simulink model "PID_Controller_sim"  (R2023a)
settings: Solver=VariableStepAuto  StartTime=0.0  StopTime=20  RelTol=1e-3
values from neighbouring files (symbols this model uses):
  c = 2050    [PID_Controller.m]    (also in set_Fun.m)
  ks = 60000    [PID_Controller.m]    (also in set_Fun.m)
  kt = 362000    [PID_Controller.m]    (also in set_Fun.m)
  ms = 1173    [PID_Controller.m]    (also in set_Fun.m)
  mu = 152.1    [PID_Controller.m]    (also in set_Fun.m)
  num_y1 = num(1,:)    [PID_Controller.m]
  num_y2 = num(2,:)    [PID_Controller.m]
  num_y3 = num(3,:)    [PID_Controller.m]
undefined symbols (not defined in the file or in its folder): den
libraries: slpidlib x5
settings Model: Creator=Administrator  LastModifiedBy=Administrator

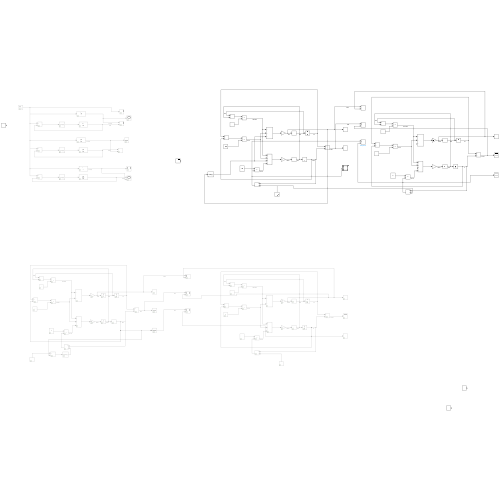
[thumbnail: Simulink's stored preview of the top-level diagram]
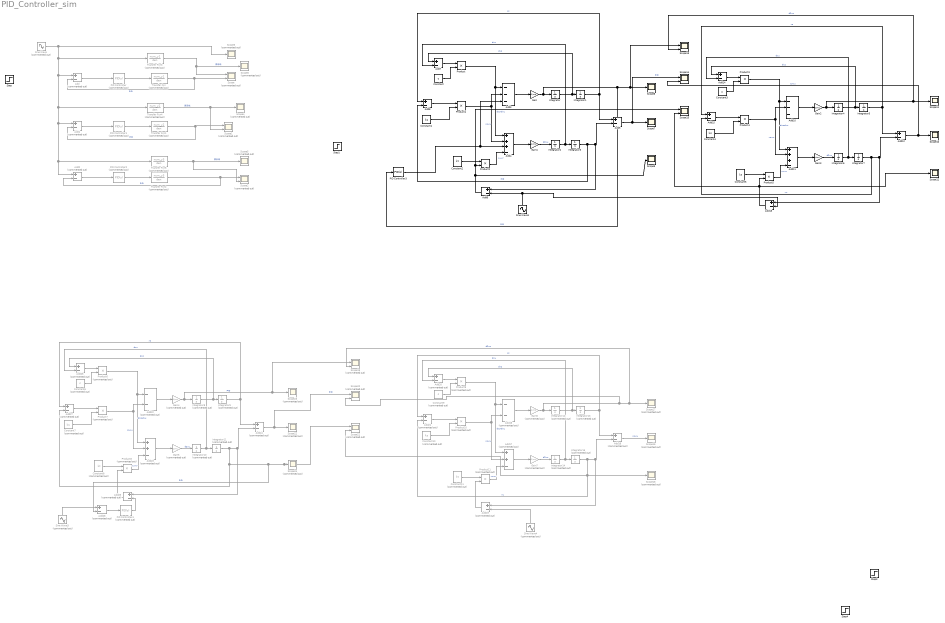
== system PID_Controller_sim ==
  Add{,1..2,18..21,24..28} (12 alike) : Sum  Commented=on  Inputs=+-
  Add10 : Sum  Inputs=---
  Add11 : Sum  Inputs=+++-
  Add{5..8,12..15} (8 alike) : Sum  Inputs=+-
  Add16 : Sum  Commented=on  Inputs=--
  Add17 : Sum  Commented=on  Inputs=++-
  Add22 : Sum  Commented=on  Inputs=--
  Add23 : Sum  Commented=on  Inputs=++-
  Add3 : Sum  Inputs=---
  Add4 : Sum  Inputs=+++-
  Constant : Constant  Value=c
  Constant1 : Constant  Value=ks
  Constant10 : Constant  Commented=on  Value=ks
  Constant11 : Constant  Commented=on  Value=kt
  Constant2 : Constant  Value=kt
  Constant3 : Constant  Value=c
  Constant4 : Constant  Value=ks
  Constant5 : Constant  Value=kt
  Constant6 : Constant  Commented=on  Value=c
  Constant7 : Constant  Commented=on  Value=ks
  Constant8 : Constant  Commented=on  Value=kt
  Constant9 : Constant  Commented=on  Value=c
  Gain : Gain  Gain=1/ms
  Gain1 : Gain  Gain=1/mu
  Gain2 : Gain  Gain=1/ms
  Gain3 : Gain  Gain=1/mu
  Gain4 : Gain  Commented=on  Gain=1/ms
  Gain5 : Gain  Commented=on  Gain=1/mu
  Gain6 : Gain  Commented=on  Gain=1/ms
  Gain7 : Gain  Commented=on  Gain=1/mu
  Integrator{,1..7} (8 alike) : Integrator
  Integrator{8..15} (8 alike) : Integrator  Commented=on
  PID Controller : slpidlib/PID Controller  Commented=on  Controller=PID  Form=Parallel  TimeDomain=Continuous-time  UseExternalTs=off  SampleTime=-1  IntegratorMethod=Forward Euler  FilterMethod=Forward Euler  ControllerParametersSource=internal  P=0.544393537633049  I=228.313262527094  UseKiTs=off  D=4.11995694275818e-05  N=8640.6528392362  UseFilter=on  TunerSelectOption=Transfer Function Based (PID Tuner App)  InitialConditionSource=internal  InitialConditionForIntegrator=0  InitialConditionForFilter=0  DifferentiatorICPrevScaledInput=0  ExternalReset=none  TrackingMode=off  Kt=1  LimitOutput=off  SatLimitsSource=internal  UpperSaturationLimit=inf  LowerSaturationLimit=-inf  LinearizeAsGain=on  AntiWindupMode=none  Kb=1  LimitIntegrator=off  UpperIntegratorSaturationLimit=inf  LowerIntegratorSaturationLimit=-inf  POutMin=[]  POutMax=[]  IOutMin=[]  IOutMax=[]  DOutMin=[]  DOutMax=[]  NOutMin=[]  NOutMax=[]  SumOutMin=[]  SumOutMax=[]  SaturationOutMin=[]  SaturationOutMax=[]  PParamMin=[]  PParamMax=[]  IParamMin=[]  IParamMax=[]  DParamMin=[]  DParamMax=[]  NParamMin=[]  NParamMax=[]  KbParamMin=[]  KbParamMax=[]  KtParamMin=[]  KtParamMax=[]  KbOutMin=[]  KbOutMax=[]  KtOutMin=[]  KtOutMax=[]  IntegratorOutMin=[]  IntegratorOutMax=[]  FilterOutMin=[]  FilterOutMax=[]  SumI1OutMin=[]  SumI1OutMax=[]  SumI2OutMin=[]  SumI2OutMax=[]  SumI3OutMin=[]  SumI3OutMax=[]  SumI4OutMin=[]  SumI4OutMax=[]  SumDOutMin=[]  SumDOutMax=[]  DifferentiatorOutMin=[]  DifferentiatorOutMax=[]  FilterDiffOutCoefMin=[]  FilterDiffOutCoefMax=[]  ReciprocalOutMin=[]  ReciprocalOutMax=[]  SumDenOutMin=[]  SumDenOutMax=[]  SumNumOutMin=[]  SumNumOutMax=[]  DivideOutMin=[]  DivideOutMax=[]  UdiffTsProdOutMin=[]  UdiffTsProdOutMax=[]  NTsProdOutMin=[]  NTsProdOutMax=[]  UintegralTsProdOutMin=[]  UintegralTsProdOutMax=[]  UngainTsProdOutMin=[]  UngainTsProdOutMax=[]  ClampingZeroOutDataTypeStr=Inherit: Inherit via back propagation  ClampingZeroOutMin=[]  ClampingZeroOutMax=[]  FilterDenConstantOutDataTypeStr=Inherit: Inherit via back propagation  FilterDenConstantOutMin=[]  FilterDenConstantOutMax=[]  PCopyOutDataTypeStr=Inherit: Inherit via back propagation  PCopyOutMin=[]  PCopyOutMax=[]  NCopyOutDataTypeStr=Inherit: Inherit via back propagation  NCopyOutMin=[]  NCopyOutMax=[]  IntegratorContinuousStateAttributes=''  IntegratorStateMustResolveToSignalObject=off  IntegratorRTWStateStorageClass=Auto  FilterContinuousStateAttributes=''  FilterStateMustResolveToSignalObject=off  FilterRTWStateStorageClass=Auto  ParallelPVariant=InternalParameters  IdealPVariant=Disabled  IVariant=InternalParameters  DVariant=InternalParameters  IntegratorVariant=Continuous  SatVariant=Disabled  AWVariant=Passthrough  PCopyVariant=Disabled  TRVariant=Disabled  FdbkBlocksVariant=Forward  IdealPFdbkVariant=Disabled  SatFdbkVariant=Disabled  DerivativeFilterVariant=ContFilter  NVariant=InternalParameters  NCopyVariant=Disabled  FilterICVariant=InternalICsFilter  IntegratorICVariant=InternalICs  ExternalResetVariant=Disabled  TRSumVariant=Passthrough  SumFdbkVariant=Disabled  SumVariant=Sum_PID  TsampFilterVariant=InternalTs  TsampNgainVariant=Passthrough  TsampIntegralVariant=Disabled_SignalSpec  ExternalSaturationOutDataTypeStr=Inherit: Same as second input
  PID Controller1 : slpidlib/PID Controller  Commented=on  Controller=PID  Form=Parallel  TimeDomain=Continuous-time  UseExternalTs=off  SampleTime=-1  IntegratorMethod=Forward Euler  FilterMethod=Forward Euler  ControllerParametersSource=internal  P=-344.974819520367  I=-34693.2038324327  UseKiTs=off  D=-0.842159264151759  N=11254.9743438156  UseFilter=on  TunerSelectOption=Transfer Function Based (PID Tuner App)  InitialConditionSource=internal  InitialConditionForIntegrator=0  InitialConditionForFilter=0  DifferentiatorICPrevScaledInput=0  ExternalReset=none  TrackingMode=off  Kt=1  LimitOutput=off  SatLimitsSource=internal  UpperSaturationLimit=inf  LowerSaturationLimit=-inf  LinearizeAsGain=on  AntiWindupMode=none  Kb=1  LimitIntegrator=off  UpperIntegratorSaturationLimit=inf  LowerIntegratorSaturationLimit=-inf  POutMin=[]  POutMax=[]  IOutMin=[]  IOutMax=[]  DOutMin=[]  DOutMax=[]  NOutMin=[]  NOutMax=[]  SumOutMin=[]  SumOutMax=[]  SaturationOutMin=[]  SaturationOutMax=[]  PParamMin=[]  PParamMax=[]  IParamMin=[]  IParamMax=[]  DParamMin=[]  DParamMax=[]  NParamMin=[]  NParamMax=[]  KbParamMin=[]  KbParamMax=[]  KtParamMin=[]  KtParamMax=[]  KbOutMin=[]  KbOutMax=[]  KtOutMin=[]  KtOutMax=[]  IntegratorOutMin=[]  IntegratorOutMax=[]  FilterOutMin=[]  FilterOutMax=[]  SumI1OutMin=[]  SumI1OutMax=[]  SumI2OutMin=[]  SumI2OutMax=[]  SumI3OutMin=[]  SumI3OutMax=[]  SumI4OutMin=[]  SumI4OutMax=[]  SumDOutMin=[]  SumDOutMax=[]  DifferentiatorOutMin=[]  DifferentiatorOutMax=[]  FilterDiffOutCoefMin=[]  FilterDiffOutCoefMax=[]  ReciprocalOutMin=[]  ReciprocalOutMax=[]  SumDenOutMin=[]  SumDenOutMax=[]  SumNumOutMin=[]  SumNumOutMax=[]  DivideOutMin=[]  DivideOutMax=[]  UdiffTsProdOutMin=[]  UdiffTsProdOutMax=[]  NTsProdOutMin=[]  NTsProdOutMax=[]  UintegralTsProdOutMin=[]  UintegralTsProdOutMax=[]  UngainTsProdOutMin=[]  UngainTsProdOutMax=[]  ClampingZeroOutDataTypeStr=Inherit: Inherit via back propagation  ClampingZeroOutMin=[]  ClampingZeroOutMax=[]  FilterDenConstantOutDataTypeStr=Inherit: Inherit via back propagation  FilterDenConstantOutMin=[]  FilterDenConstantOutMax=[]  PCopyOutDataTypeStr=Inherit: Inherit via back propagation  PCopyOutMin=[]  PCopyOutMax=[]  NCopyOutDataTypeStr=Inherit: Inherit via back propagation  NCopyOutMin=[]  NCopyOutMax=[]  IntegratorContinuousStateAttributes=''  IntegratorStateMustResolveToSignalObject=off  IntegratorRTWStateStorageClass=Auto  FilterContinuousStateAttributes=''  FilterStateMustResolveToSignalObject=off  FilterRTWStateStorageClass=Auto  ParallelPVariant=InternalParameters  IdealPVariant=Disabled  IVariant=InternalParameters  DVariant=InternalParameters  IntegratorVariant=Continuous  SatVariant=Disabled  AWVariant=Passthrough  PCopyVariant=Disabled  TRVariant=Disabled  FdbkBlocksVariant=Forward  IdealPFdbkVariant=Disabled  SatFdbkVariant=Disabled  DerivativeFilterVariant=ContFilter  NVariant=InternalParameters  NCopyVariant=Disabled  FilterICVariant=InternalICsFilter  IntegratorICVariant=InternalICs  ExternalResetVariant=Disabled  TRSumVariant=Passthrough  SumFdbkVariant=Disabled  SumVariant=Sum_PID  TsampFilterVariant=InternalTs  TsampNgainVariant=Passthrough  TsampIntegralVariant=Disabled_SignalSpec  ExternalSaturationOutDataTypeStr=Inherit: Same as second input
  PID Controller2 : slpidlib/PID Controller  Commented=on  Controller=PID  Form=Parallel  TimeDomain=Continuous-time  UseExternalTs=off  SampleTime=-1  IntegratorMethod=Forward Euler  FilterMethod=Forward Euler  ControllerParametersSource=internal  P=11.2600420001673  I=219.670632938748  UseKiTs=off  D=0.100649946633639  N=30187.8390185077  UseFilter=on  TunerSelectOption=Transfer Function Based (PID Tuner App)  InitialConditionSource=internal  InitialConditionForIntegrator=0  InitialConditionForFilter=0  DifferentiatorICPrevScaledInput=0  ExternalReset=none  TrackingMode=off  Kt=1  LimitOutput=off  SatLimitsSource=internal  UpperSaturationLimit=inf  LowerSaturationLimit=-inf  LinearizeAsGain=on  AntiWindupMode=none  Kb=1  LimitIntegrator=off  UpperIntegratorSaturationLimit=inf  LowerIntegratorSaturationLimit=-inf  POutMin=[]  POutMax=[]  IOutMin=[]  IOutMax=[]  DOutMin=[]  DOutMax=[]  NOutMin=[]  NOutMax=[]  SumOutMin=[]  SumOutMax=[]  SaturationOutMin=[]  SaturationOutMax=[]  PParamMin=[]  PParamMax=[]  IParamMin=[]  IParamMax=[]  DParamMin=[]  DParamMax=[]  NParamMin=[]  NParamMax=[]  KbParamMin=[]  KbParamMax=[]  KtParamMin=[]  KtParamMax=[]  KbOutMin=[]  KbOutMax=[]  KtOutMin=[]  KtOutMax=[]  IntegratorOutMin=[]  IntegratorOutMax=[]  FilterOutMin=[]  FilterOutMax=[]  SumI1OutMin=[]  SumI1OutMax=[]  SumI2OutMin=[]  SumI2OutMax=[]  SumI3OutMin=[]  SumI3OutMax=[]  SumI4OutMin=[]  SumI4OutMax=[]  SumDOutMin=[]  SumDOutMax=[]  DifferentiatorOutMin=[]  DifferentiatorOutMax=[]  FilterDiffOutCoefMin=[]  FilterDiffOutCoefMax=[]  ReciprocalOutMin=[]  ReciprocalOutMax=[]  SumDenOutMin=[]  SumDenOutMax=[]  SumNumOutMin=[]  SumNumOutMax=[]  DivideOutMin=[]  DivideOutMax=[]  UdiffTsProdOutMin=[]  UdiffTsProdOutMax=[]  NTsProdOutMin=[]  NTsProdOutMax=[]  UintegralTsProdOutMin=[]  UintegralTsProdOutMax=[]  UngainTsProdOutMin=[]  UngainTsProdOutMax=[]  ClampingZeroOutDataTypeStr=Inherit: Inherit via back propagation  ClampingZeroOutMin=[]  ClampingZeroOutMax=[]  FilterDenConstantOutDataTypeStr=Inherit: Inherit via back propagation  FilterDenConstantOutMin=[]  FilterDenConstantOutMax=[]  PCopyOutDataTypeStr=Inherit: Inherit via back propagation  PCopyOutMin=[]  PCopyOutMax=[]  NCopyOutDataTypeStr=Inherit: Inherit via back propagation  NCopyOutMin=[]  NCopyOutMax=[]  IntegratorContinuousStateAttributes=''  IntegratorStateMustResolveToSignalObject=off  IntegratorRTWStateStorageClass=Auto  FilterContinuousStateAttributes=''  FilterStateMustResolveToSignalObject=off  FilterRTWStateStorageClass=Auto  ParallelPVariant=InternalParameters  IdealPVariant=Disabled  IVariant=InternalParameters  DVariant=InternalParameters  IntegratorVariant=Continuous  SatVariant=Disabled  AWVariant=Passthrough  PCopyVariant=Disabled  TRVariant=Disabled  FdbkBlocksVariant=Forward  IdealPFdbkVariant=Disabled  SatFdbkVariant=Disabled  DerivativeFilterVariant=ContFilter  NVariant=InternalParameters  NCopyVariant=Disabled  FilterICVariant=InternalICsFilter  IntegratorICVariant=InternalICs  ExternalResetVariant=Disabled  TRSumVariant=Passthrough  SumFdbkVariant=Disabled  SumVariant=Sum_PID  TsampFilterVariant=InternalTs  TsampNgainVariant=Passthrough  TsampIntegralVariant=Disabled_SignalSpec  ExternalSaturationOutDataTypeStr=Inherit: Same as second input
  PID Controller3 : slpidlib/PID Controller  Controller=PID  Form=Parallel  TimeDomain=Continuous-time  UseExternalTs=off  SampleTime=-1  IntegratorMethod=Forward Euler  FilterMethod=Forward Euler  ControllerParametersSource=internal  P=1000  I=6000  UseKiTs=off  D=100  N=200  UseFilter=on  TunerSelectOption=Transfer Function Based (PID Tuner App)  InitialConditionSource=internal  InitialConditionForIntegrator=0  InitialConditionForFilter=0  DifferentiatorICPrevScaledInput=0  ExternalReset=none  TrackingMode=off  Kt=1  LimitOutput=off  SatLimitsSource=internal  UpperSaturationLimit=inf  LowerSaturationLimit=-inf  LinearizeAsGain=on  AntiWindupMode=none  Kb=1  LimitIntegrator=off  UpperIntegratorSaturationLimit=inf  LowerIntegratorSaturationLimit=-inf  POutMin=[]  POutMax=[]  IOutMin=[]  IOutMax=[]  DOutMin=[]  DOutMax=[]  NOutMin=[]  NOutMax=[]  SumOutMin=[]  SumOutMax=[]  SaturationOutMin=[]  SaturationOutMax=[]  PParamMin=[]  PParamMax=[]  IParamMin=[]  IParamMax=[]  DParamMin=[]  DParamMax=[]  NParamMin=[]  NParamMax=[]  KbParamMin=[]  KbParamMax=[]  KtParamMin=[]  KtParamMax=[]  KbOutMin=[]  KbOutMax=[]  KtOutMin=[]  KtOutMax=[]  IntegratorOutMin=[]  IntegratorOutMax=[]  FilterOutMin=[]  FilterOutMax=[]  SumI1OutMin=[]  SumI1OutMax=[]  SumI2OutMin=[]  SumI2OutMax=[]  SumI3OutMin=[]  SumI3OutMax=[]  SumI4OutMin=[]  SumI4OutMax=[]  SumDOutMin=[]  SumDOutMax=[]  DifferentiatorOutMin=[]  DifferentiatorOutMax=[]  FilterDiffOutCoefMin=[]  FilterDiffOutCoefMax=[]  ReciprocalOutMin=[]  ReciprocalOutMax=[]  SumDenOutMin=[]  SumDenOutMax=[]  SumNumOutMin=[]  SumNumOutMax=[]  DivideOutMin=[]  DivideOutMax=[]  UdiffTsProdOutMin=[]  UdiffTsProdOutMax=[]  NTsProdOutMin=[]  NTsProdOutMax=[]  UintegralTsProdOutMin=[]  UintegralTsProdOutMax=[]  UngainTsProdOutMin=[]  UngainTsProdOutMax=[]  ClampingZeroOutDataTypeStr=Inherit: Inherit via back propagation  ClampingZeroOutMin=[]  ClampingZeroOutMax=[]  FilterDenConstantOutDataTypeStr=Inherit: Inherit via back propagation  FilterDenConstantOutMin=[]  FilterDenConstantOutMax=[]  PCopyOutDataTypeStr=Inherit: Inherit via back propagation  PCopyOutMin=[]  PCopyOutMax=[]  NCopyOutDataTypeStr=Inherit: Inherit via back propagation  NCopyOutMin=[]  NCopyOutMax=[]  IntegratorContinuousStateAttributes=''  IntegratorStateMustResolveToSignalObject=off  IntegratorRTWStateStorageClass=Auto  FilterContinuousStateAttributes=''  FilterStateMustResolveToSignalObject=off  FilterRTWStateStorageClass=Auto  ParallelPVariant=InternalParameters  IdealPVariant=Disabled  IVariant=InternalParameters  DVariant=InternalParameters  IntegratorVariant=Continuous  SatVariant=Disabled  AWVariant=Passthrough  PCopyVariant=Disabled  TRVariant=Disabled  FdbkBlocksVariant=Forward  IdealPFdbkVariant=Disabled  SatFdbkVariant=Disabled  DerivativeFilterVariant=ContFilter  NVariant=InternalParameters  NCopyVariant=Disabled  FilterICVariant=InternalICsFilter  IntegratorICVariant=InternalICs  ExternalResetVariant=Disabled  TRSumVariant=Passthrough  SumFdbkVariant=Disabled  SumVariant=Sum_PID  TsampFilterVariant=InternalTs  TsampNgainVariant=Passthrough  TsampIntegralVariant=Disabled_SignalSpec  ExternalSaturationOutDataTypeStr=Inherit: Same as second input
  PID Controller4 : slpidlib/PID Controller  Commented=on  Controller=PID  Form=Parallel  TimeDomain=Continuous-time  UseExternalTs=off  SampleTime=-1  IntegratorMethod=Forward Euler  FilterMethod=Forward Euler  ControllerParametersSource=internal  P=10.0881443003307  I=160.158802692204  UseKiTs=off  D=0.156139383823636  N=43634.7031102267  UseFilter=on  TunerSelectOption=Transfer Function Based (PID Tuner App)  InitialConditionSource=internal  InitialConditionForIntegrator=0  InitialConditionForFilter=0  DifferentiatorICPrevScaledInput=0  ExternalReset=none  TrackingMode=off  Kt=1  LimitOutput=off  SatLimitsSource=internal  UpperSaturationLimit=inf  LowerSaturationLimit=-inf  LinearizeAsGain=on  AntiWindupMode=none  Kb=1  LimitIntegrator=off  UpperIntegratorSaturationLimit=inf  LowerIntegratorSaturationLimit=-inf  POutMin=[]  POutMax=[]  IOutMin=[]  IOutMax=[]  DOutMin=[]  DOutMax=[]  NOutMin=[]  NOutMax=[]  SumOutMin=[]  SumOutMax=[]  SaturationOutMin=[]  SaturationOutMax=[]  PParamMin=[]  PParamMax=[]  IParamMin=[]  IParamMax=[]  DParamMin=[]  DParamMax=[]  NParamMin=[]  NParamMax=[]  KbParamMin=[]  KbParamMax=[]  KtParamMin=[]  KtParamMax=[]  KbOutMin=[]  KbOutMax=[]  KtOutMin=[]  KtOutMax=[]  IntegratorOutMin=[]  IntegratorOutMax=[]  FilterOutMin=[]  FilterOutMax=[]  SumI1OutMin=[]  SumI1OutMax=[]  SumI2OutMin=[]  SumI2OutMax=[]  SumI3OutMin=[]  SumI3OutMax=[]  SumI4OutMin=[]  SumI4OutMax=[]  SumDOutMin=[]  SumDOutMax=[]  DifferentiatorOutMin=[]  DifferentiatorOutMax=[]  FilterDiffOutCoefMin=[]  FilterDiffOutCoefMax=[]  ReciprocalOutMin=[]  ReciprocalOutMax=[]  SumDenOutMin=[]  SumDenOutMax=[]  SumNumOutMin=[]  SumNumOutMax=[]  DivideOutMin=[]  DivideOutMax=[]  UdiffTsProdOutMin=[]  UdiffTsProdOutMax=[]  NTsProdOutMin=[]  NTsProdOutMax=[]  UintegralTsProdOutMin=[]  UintegralTsProdOutMax=[]  UngainTsProdOutMin=[]  UngainTsProdOutMax=[]  ClampingZeroOutDataTypeStr=Inherit: Inherit via back propagation  ClampingZeroOutMin=[]  ClampingZeroOutMax=[]  FilterDenConstantOutDataTypeStr=Inherit: Inherit via back propagation  FilterDenConstantOutMin=[]  FilterDenConstantOutMax=[]  PCopyOutDataTypeStr=Inherit: Inherit via back propagation  PCopyOutMin=[]  PCopyOutMax=[]  NCopyOutDataTypeStr=Inherit: Inherit via back propagation  NCopyOutMin=[]  NCopyOutMax=[]  IntegratorContinuousStateAttributes=''  IntegratorStateMustResolveToSignalObject=off  IntegratorRTWStateStorageClass=Auto  FilterContinuousStateAttributes=''  FilterStateMustResolveToSignalObject=off  FilterRTWStateStorageClass=Auto  ParallelPVariant=InternalParameters  IdealPVariant=Disabled  IVariant=InternalParameters  DVariant=InternalParameters  IntegratorVariant=Continuous  SatVariant=Disabled  AWVariant=Passthrough  PCopyVariant=Disabled  TRVariant=Disabled  FdbkBlocksVariant=Forward  IdealPFdbkVariant=Disabled  SatFdbkVariant=Disabled  DerivativeFilterVariant=ContFilter  NVariant=InternalParameters  NCopyVariant=Disabled  FilterICVariant=InternalICsFilter  IntegratorICVariant=InternalICs  ExternalResetVariant=Disabled  TRSumVariant=Passthrough  SumFdbkVariant=Disabled  SumVariant=Sum_PID  TsampFilterVariant=InternalTs  TsampNgainVariant=Passthrough  TsampIntegralVariant=Disabled_SignalSpec  ExternalSaturationOutDataTypeStr=Inherit: Same as second input
  Product{,1..5} (6 alike) : Product
  Product{6..11} (6 alike) : Product  Commented=on
  Scope{,1..2,19..21} (6 alike) : Scope  Commented=on  NumInputPorts=2
  Scope{7..12} (6 alike) : Scope
  Scope13 : Scope  NumInputPorts=2
  Scope14 : Scope  NumInputPorts=2
  Scope15 : Scope  NumInputPorts=2
  Scope{3..6,16..18,22..24} (10 alike) : Scope  Commented=on
  Sine Wave : Sin  Commented=on  SampleTime=0
  Sine Wave1 : Sin  Amplitude=0.05  Frequency=2*pi  SampleTime=0
  Sine Wave3 : Sin  Commented=on  Amplitude=0.1  SampleTime=0
  Sine Wave4 : Sin  Commented=on  Amplitude=0.1  SampleTime=0
  Step : Step  SampleTime=0
  Step1 : Step  Time=0.1  SampleTime=0
  Step3 : Step  Time=0.1  SampleTime=0
  Step4 : Step  Time=0.1  SampleTime=0
  Transfer Fcn : TransferFcn  Commented=on  Numerator=num_y1  Denominator=den
  Transfer Fcn1 : TransferFcn  Commented=on  Numerator=num_y2  Denominator=den
  Transfer Fcn2 : TransferFcn  Commented=on  Numerator=num_y3  Denominator=den
  Transfer Fcn3 : TransferFcn  Commented=on  Numerator=num_y1  Denominator=den
  Transfer Fcn4 : TransferFcn  Commented=on  Numerator=num_y2  Denominator=den
  Transfer Fcn5 : TransferFcn  Commented=on  Numerator=num_y3  Denominator=den
  wires:
  Sine Wave/1 -> Transfer Fcn4/1, Transfer Fcn5/1, Add2/1, Add1/1, Add/1, Transfer Fcn3/1, Scope3/1
  Add/1 -> PID Controller/1
  PID Controller/1 -> Transfer Fcn/1
  Transfer Fcn/1 -> Add/2, Scope/2  "PID"
  Transfer Fcn3/1 -> Scope6/1, Scope/1  "原系统"
  PID Controller1/1 -> Transfer Fcn1/1
  Add1/1 -> PID Controller1/1
  Transfer Fcn1/1 -> Add1/2, Scope1/1  "PID"
  PID Controller2/1 -> Transfer Fcn2/1
  Add2/1 -> PID Controller2/1
  Transfer Fcn2/1 -> Add2/2, Scope2/1  "PID"
  Transfer Fcn4/1 -> Scope1/2, Scope4/1  "原系统"
  Transfer Fcn5/1 -> Scope5/1, Scope2/2  "原系统"
  Add3/1 -> Gain/1
  Add4/1 -> Gain1/1
  Gain/1 -> PID Controller3/1, Scope13/1, Scope8/1, Integrator/1  "PID"
  Integrator/1 -> Add7/1, Integrator1/1  "dxs"
  Gain1/1 -> Integrator2/1  "d2xu"
  Integrator2/1 -> Add7/2, Integrator3/1  "dxu"
  Integrator1/1 -> Add5/1, Add8/1  "xs"
  Integrator3/1 -> Add8/2, Add6/1, Add5/2  "PID"
  Add5/1 -> Scope14/1, Scope7/1  "PID"
  Constant/1 -> Product/2
  Constant1/1 -> Product1/2
  Constant2/1 -> Product2/1
  Product2/1 -> Add4/4  "xu-xr"
  Product/1 -> Add4/1, Add3/1  "dxs-dxu"
  Product1/1 -> Add4/2, Add3/2  "xs-xu"
  PID Controller3/1 -> Add3/3, Add4/3
  Add7/1 -> Product/1
  Add8/1 -> Product1/1
  Sine Wave1/1 -> Add6/2, Add13/2
  Integrator4/1 -> Add14/1, Integrator5/1  "dxs"
  Add10/1 -> Gain2/1
  Integrator6/1 -> Add14/2, Integrator7/1  "dxu"
  Product4/1 -> Add11/2, Add10/2  "xs-xu"
  Gain2/1 -> Scope13/2, Scope11/1, Integrator4/1  "d2xs"
  Constant5/1 -> Product5/1
  Gain3/1 -> Integrator6/1  "d2xu"
  Integrator7/1 -> Add15/2, Add13/1, Add12/2  "xu"
  Add14/1 -> Product3/1
  Add11/1 -> Gain3/1
  Product5/1 -> Add11/4  "xu-xr"
  Constant4/1 -> Product4/2
  Constant3/1 -> Product3/2
  Product3/1 -> Add11/1, Add10/1  "dxs-dxu"
  Add15/1 -> Product4/1
  Add12/1 -> Scope14/2, Scope10/1  "xs-xu"
  Integrator5/1 -> Add12/1, Add15/1  "xs"
  Add23/1 -> Gain5/1
  Constant11/1 -> Product11/1
  Add18/1 -> Scope16/1  "xs-xu"
  Product10/1 -> Add17/2, Add16/2  "xs-xu"
  Constant8/1 -> Product8/1
  Add21/1 -> Product10/1
  Integrator15/1 -> Scope18/1, Scope21/2, Add21/2, Add19/1, Add18/2  "xu"
  Integrator11/1 -> Add27/2, Add28/2, Scope21/1, Scope24/1, Add25/1, Add24/2  "PID"
  Add20/1 -> Product9/1
  Integrator12/1 -> Add20/1, Integrator13/1  "dxs"
  Constant9/1 -> Product9/2
  Sine Wave3/1 -> Add28/1
  Add27/1 -> Product7/1
  Gain7/1 -> Integrator14/1  "d2xu"
  Gain6/1 -> Scope20/2, Scope19/2, Scope17/1, Integrator12/1  "d2xs"
  Add24/1 -> Scope22/1, Scope20/1  "PID"
  Add19/1 -> Product11/2
  Constant10/1 -> Product10/2
  Gain4/1 -> Scope19/1, Scope23/1, Integrator8/1  "PID"
  Product7/1 -> Add23/2, Add22/2  "xs-xu"
  Add28/1 -> PID Controller4/1
  Add26/1 -> Product6/1
  Add16/1 -> Gain6/1
  Add25/1 -> Product8/2
  Integrator14/1 -> Add20/2, Integrator15/1  "dxu"
  Sine Wave4/1 -> Add19/2
  Product11/1 -> Add17/3  "xu-xr"
  Constant7/1 -> Product7/2
  Gain5/1 -> Integrator10/1  "d2xu"
  Integrator8/1 -> Add26/1, Integrator9/1  "dxs"
  Product8/1 -> Add23/3  "xu-xr"
  Product9/1 -> Add17/1, Add16/1  "dxs-dxu"
  Constant6/1 -> Product6/2
  Add17/1 -> Gain7/1
  Add22/1 -> Gain4/1
  Integrator9/1 -> Add24/1, Add27/1  "xs"
  Product6/1 -> Add23/1, Add22/1  "dxs-dxu"
  Integrator10/1 -> Add26/2, Integrator11/1  "dxu"
  Integrator13/1 -> Add18/1, Add21/1  "xs"
  PID Controller4/1 -> Add25/2
  Add13/1 -> Product5/2, Scope15/2, Scope12/1
  Add6/1 -> Scope15/1, Product2/2, Scope9/1
